simulink model "sharedControl3"  (R2018a)
settings: Solver=FixedStepAuto  StartTime=0.0  StopTime=500  FixedStep=.1  RelTol=1e-3
libraries: commfilt2 x2, simulink x2
settings Model: Creator=transmogrifierlight  LastModifiedBy=transmogrifier

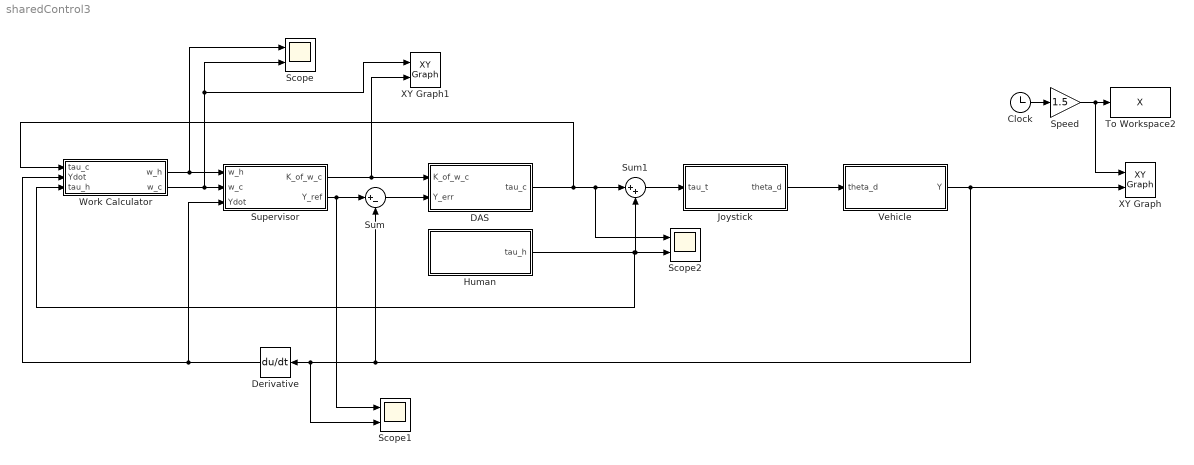
== system sharedControl3 ==
  Clock : Clock
  DAS : Subsystem
  Derivative : Derivative
  Human : Subsystem
  Joystick : Subsystem
  Scope : Scope  NumInputPorts=2
  Scope1 : Scope  NumInputPorts=2
  Scope2 : Scope  NumInputPorts=2
  Speed : Gain  Gain=1.5
  Sum : Sum  Inputs=|+-
  Sum1 : Sum  Inputs=|++
  Supervisor : Subsystem  mask{gamma_1_sq=0.1, gamma_2_sq=0.2, a_d=10, b_d=0.4, sigma_sq=0.3, delta_y=4, K0=0.5}
      mask prompts: gamma_1_sq "DAS Threshold"; gamma_2_sq "Human Threshold"; a_d "a"; b_d "b"; sigma_sq "Lane Change Threshold"; delta_y "Lane Change Delta"
  To Workspace2 : ToWorkspace  VariableName=X  SaveFormat=Timeseries  SampleTime=-1
  Vehicle : Subsystem
  Work Calculator : Subsystem
  XY Graph : simulink/Sinks/XY Graph  xmin=-10  xmax=1.5*1500  ymin=-100  ymax=100  st=-1
  XY Graph1 : simulink/Sinks/XY Graph  xmin=-01  xmax=2  ymin=-0.5  ymax=1  st=-1
  wires:
  Work Calculator/1(w_h) -> Scope/1, Supervisor/1(w_h)
  Work Calculator/2(w_c) -> XY Graph1/1, Scope/2, Supervisor/2(w_c)
  Supervisor/1(K_of_w_c) -> XY Graph1/2, DAS/1("K_of_w_c ")
  Supervisor/2(Y_ref) -> Scope1/1, Sum/1
  Sum/1 -> DAS/2(Y_err)
  DAS/1(tau_c) -> Scope2/1, Sum1/1, Work Calculator/1(tau_c)
  Sum1/1 -> Joystick/1(tau_t)
  Clock/1 -> Speed/1
  Speed/1 -> XY Graph/1, To Workspace2/1
  Vehicle/1(Y) -> Sum/2, Scope1/2, Derivative/1, XY Graph/2
  Derivative/1 -> Supervisor/3(Ydot), Work Calculator/2(Ydot)
  Joystick/1(theta_d) -> Vehicle/1(theta_d)
  Human/1(tau_h) -> Work Calculator/3(tau_h), Sum1/2, Scope2/2

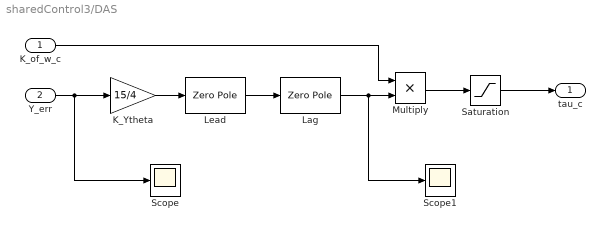
== system sharedControl3/DAS ==
  "K_of_w_c " : Inport
  Y_err : Inport  Port=2
  K_Ytheta : Gain  Gain=15/4
  Lag : ZeroPole  Zeros=[-0.0889]  Poles=[-0.0022]
  Lead : ZeroPole  Zeros=[-0.4]  Poles=[-26.7354]  Gain=[469.1235]
  Multiply : Product
  Saturation : Saturate  UpperLimit=3.5  LowerLimit=-3.5
  Scope : Scope
  Scope1 : Scope
  tau_c : Outport
  wires:
  Y_err/1 -> Scope/1, K_Ytheta/1
  Saturation/1 -> tau_c/1
  Multiply/1 -> Saturation/1
  "K_of_w_c "/1 -> Multiply/1
  K_Ytheta/1 -> Lead/1
  Lead/1 -> Lag/1
  Lag/1 -> Scope1/1, Multiply/2

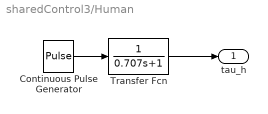
== system sharedControl3/Human ==
  Continuous Pulse Generator : DiscretePulseGenerator  PulseType=Time based  Amplitude=3.5  Period=100  PhaseDelay=30
  Transfer Fcn : TransferFcn  Denominator=[0.707 1]
  tau_h : Outport
  wires:
  Transfer Fcn/1 -> tau_h/1
  Continuous Pulse Generator/1 -> Transfer Fcn/1

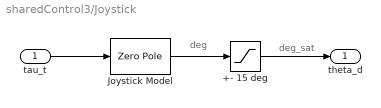
== system sharedControl3/Joystick ==
  note: deg_sat
  note: deg
  tau_t : Inport
  +- 15 deg : Saturate  UpperLimit=15  LowerLimit=-15
  Joystick Model : ZeroPole  Zeros=[]  Poles=[0 -0.254/0.762]  Gain=[0.762]
  theta_d : Outport
  wires:
  Joystick Model/1 -> +- 15 deg/1
  +- 15 deg/1 -> theta_d/1
  tau_t/1 -> Joystick Model/1

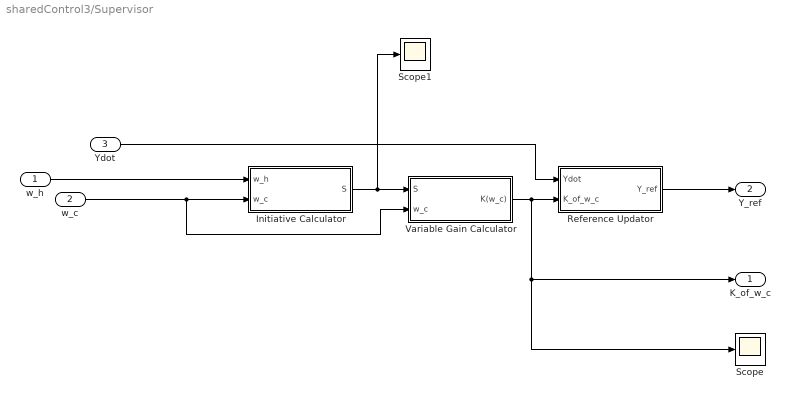
== system sharedControl3/Supervisor ==
  w_h : Inport
  w_c : Inport  Port=2
  Ydot : Inport  Port=3
  Initiative Calculator : Subsystem
  Reference Updator : Subsystem
  Scope : Scope
  Scope1 : Scope
  Variable Gain Calculator : Subsystem
  K_of_w_c : Outport
  Y_ref : Outport  Port=2
  wires:
  w_c/1 -> Variable Gain Calculator/2(w_c), Initiative Calculator/2("w_c ")
  w_h/1 -> Initiative Calculator/1(w_h)
  Initiative Calculator/1(S) -> Scope1/1, Variable Gain Calculator/1(S)
  Variable Gain Calculator/1(K(w_c)) -> Reference Updator/2(K_of_w_c), Scope/1, K_of_w_c/1
  Ydot/1 -> Reference Updator/1(Ydot)
  Reference Updator/1(Y_ref) -> Y_ref/1

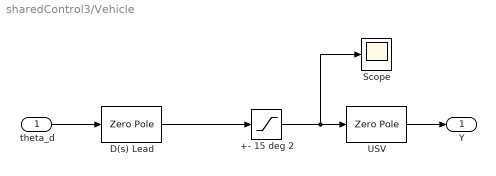
== system sharedControl3/Vehicle ==
  theta_d : Inport
  +- 15 deg 2 : Saturate  UpperLimit=15  LowerLimit=-15
  D(s) Lead : ZeroPole  Zeros=[-.2667]  Poles=[-26.49]  Gain=[1619]
  Scope : Scope
  USV : ZeroPole  Zeros=[]  Poles=[0 0 -5/4]  Gain=[1.5*1e-2]
  Y : Outport
  wires:
  theta_d/1 -> D(s) Lead/1
  +- 15 deg 2/1 -> Scope/1, USV/1
  USV/1 -> Y/1
  D(s) Lead/1 -> +- 15 deg 2/1

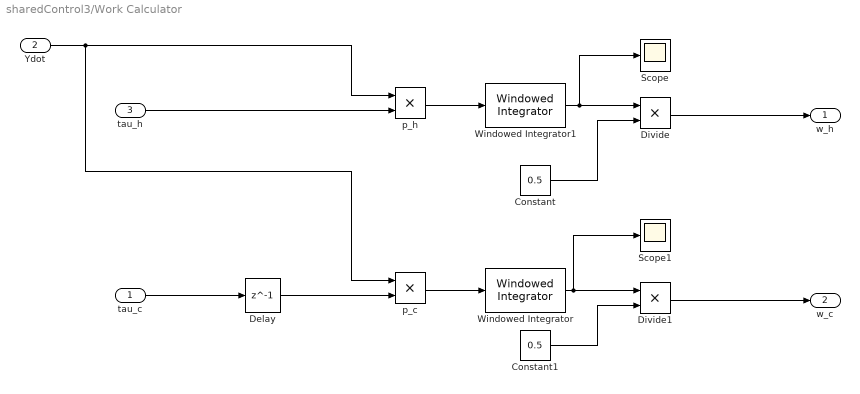
== system sharedControl3/Work Calculator ==
  tau_c : Inport
  Ydot : Inport  Port=2
  tau_h : Inport  Port=3
  Constant : Constant  Value=0.5
  Constant1 : Constant  Value=0.5
  Delay : Delay  DelayLength=1
  Divide : Product
  Divide1 : Product
  Scope : Scope
  Scope1 : Scope
  Windowed Integrator : commfilt2/Windowed Integrator  integperiod=20  InputProcessing=Columns as channels (frame based)  roundingMode=Floor  overflowMode=off  coeffDataTypeStr=Inherit: Same word length as input  coeffMin=[]  coeffMax=[]  coeffLastDataTypeStr=Inherit: Same word length as input  accumDataTypeStr=Inherit: Same as product output  accumLastDataTypeStr=Inherit: Same as product output  outputDataTypeStr=Inherit: Same as accumulator  outputMin=[]  outputMax=[]  outputLastDataTypeStr=Inherit: Same as accumulator
      settings: SourceProductName=Communications System Toolbox  SourceProductBaseCode=CM
  Windowed Integrator1 : commfilt2/Windowed Integrator  integperiod=20  InputProcessing=Columns as channels (frame based)  roundingMode=Floor  overflowMode=off  coeffDataTypeStr=Inherit: Same word length as input  coeffMin=[]  coeffMax=[]  coeffLastDataTypeStr=Inherit: Same word length as input  accumDataTypeStr=Inherit: Same as product output  accumLastDataTypeStr=Inherit: Same as product output  outputDataTypeStr=Inherit: Same as accumulator  outputMin=[]  outputMax=[]  outputLastDataTypeStr=Inherit: Same as accumulator
      settings: SourceProductName=Communications System Toolbox  SourceProductBaseCode=CM
  p_c : Product
  p_h : Product
  w_h : Outport
  w_c : Outport  Port=2
  wires:
  Divide/1 -> w_h/1
  Ydot/1 -> p_c/1, p_h/1
  Constant/1 -> Divide/2
  p_h/1 -> Windowed Integrator1/1
  tau_h/1 -> p_h/2
  tau_c/1 -> Delay/1
  Windowed Integrator/1 -> Scope1/1, Divide1/1
  p_c/1 -> Windowed Integrator/1
  Constant1/1 -> Divide1/2
  Divide1/1 -> w_c/1
  Windowed Integrator1/1 -> Scope/1, Divide/1
  Delay/1 -> p_c/2

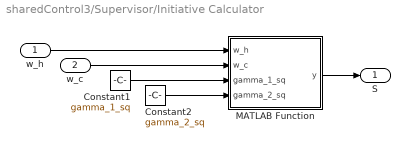
== system sharedControl3/Supervisor/Initiative Calculator ==
  w_h : Inport
  "w_c " : Inport  Port=2
  Constant1 : Constant  Value=gamma_1_sq
  Constant2 : Constant  Value=gamma_2_sq
  MATLAB Function : MATLAB Function  TreatAsAtomicUnit=on
  S : Outport
  wires:
  w_h/1 -> MATLAB Function/1(w_h)
  MATLAB Function/1(y) -> S/1
  Constant2/1 -> MATLAB Function/4(gamma_2_sq)
  "w_c "/1 -> MATLAB Function/2(w_c)
  Constant1/1 -> MATLAB Function/3(gamma_1_sq)

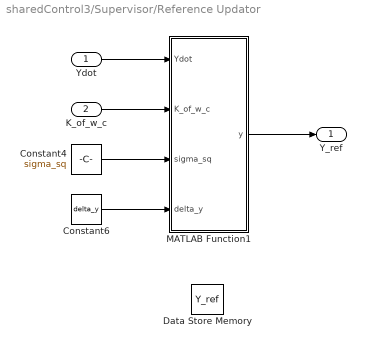
== system sharedControl3/Supervisor/Reference Updator ==
  Ydot : Inport
  K_of_w_c : Inport  Port=2
  Constant4 : Constant  Value=sigma_sq
  Constant6 : Constant  Value=delta_y
  Data Store Memory : DataStoreMemory  DataStoreName=Y_ref  ReadBeforeWriteMsg=warning  WriteAfterWriteMsg=warning  WriteAfterReadMsg=warning  ShowAdditionalParam=off  OutDataTypeStr=int16
  MATLAB Function1 : MATLAB Function  TreatAsAtomicUnit=on
  Y_ref : Outport
  wires:
  Constant4/1 -> MATLAB Function1/3(sigma_sq)
  Constant6/1 -> MATLAB Function1/4(delta_y)
  MATLAB Function1/1(y) -> Y_ref/1
  K_of_w_c/1 -> MATLAB Function1/2(K_of_w_c)
  Ydot/1 -> MATLAB Function1/1(Ydot)

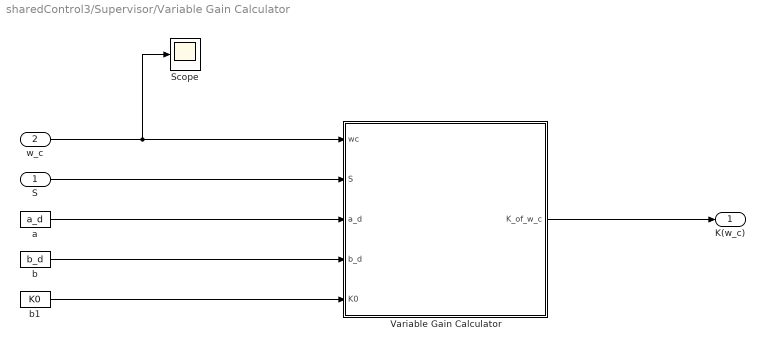
== system sharedControl3/Supervisor/Variable Gain Calculator ==
  S : Inport
  w_c : Inport  Port=2
  Scope : Scope
  "Variable Gain Calculator " : MATLAB Function  TreatAsAtomicUnit=on
  a : Constant  Value=a_d
  b : Constant  Value=b_d
  b1 : Constant  Value=K0
  K(w_c) : Outport
  wires:
  "Variable Gain Calculator "/1(K_of_w_c) -> K(w_c)/1
  a/1 -> "Variable Gain Calculator "/3(a_d)
  w_c/1 -> Scope/1, "Variable Gain Calculator "/1(wc)
  S/1 -> "Variable Gain Calculator "/2(S)
  b/1 -> "Variable Gain Calculator "/4(b_d)
  b1/1 -> "Variable Gain Calculator "/5(K0)

== matlab function sharedControl3/Supervisor/Initiative Calculator/MATLAB Function ==
  data: w_h input; y output; w_c input; gamma_1_sq input; gamma_2_sq input
function y = fcn(w_h, w_c, gamma_1_sq, gamma_2_sq)

if(w_h >= -gamma_1_sq && w_c >= -gamma_2_sq)
    S=1;
elseif(w_h >= -gamma_1_sq && w_c < -gamma_2_sq)
    S=2;
elseif(w_h < -gamma_1_sq && w_c >= -gamma_2_sq)
    S=3;
elseif(w_h < -gamma_1_sq && w_c < -gamma_2_sq)
    S=4;
else
    error('bad state assignment');
end
y = S;

== matlab function sharedControl3/Supervisor/Variable Gain Calculator/Variable Gain Calculator  ==
  data: wc input; S input; K_of_w_c output; a_d input; b_d input; K0 input
function K_of_w_c = fcn(wc, S, a_d, b_d, K0)

if S == 2    
    K_of_w_c = K0/(1 + exp(-a_d*wc + b_d));
else
    K_of_w_c = K0;
end

return

== matlab function sharedControl3/Supervisor/Reference Updator/MATLAB Function1 ==
  settings: updateMethod=DISCRETE
  data: Ydot input; y output; K_of_w_c input; sigma_sq input; delta_y input; Y_ref data_store_memory
function y = fcn(Ydot, K_of_w_c, sigma_sq, delta_y)
%Initial Y_ref, delta_y, and sigma_sq are set in mask)
disp(K_of_w_c)
global Y_ref;
if(K_of_w_c<=sigma_sq)
    if(Ydot<0)
        Y_ref=Y_ref-delta_y;
    elseif(Ydot>0)
        Y_ref=Y_ref+delta_y;
    end
end

y = Y_ref;
